simulink model "Table_airbus_v1"  (R2021b)
settings: Solver=VariableStepAuto  StartTime=0.0  StopTime=20  MaxStep=0.01  RelTol=0.01
undefined symbols (not defined in the file): X, Y, Z
libraries: sm_lib x907, fl_lib x69, nesl_utility x53, sdl_lib x10, ee_lib x7, slpidlib x6, simulink x5, simulink_extras x4
(part 17 of 18)

== system Table_airbus_v1/Modèle mécanique/Table/table_1_RIGID/x15060_M_01002_Ens_cadre_Default_1_RIGID/x15060_M_01004_Ens_barre_de_cadre_1_Default_2_RIGID/x15060_M_01042_Barre_transversale_AA_DEFAULT_1_RIGID ==
  ReferenceFrame : sm_lib/Frames and Transforms/Reference Frame
  Solid : sm_lib/Body Elements/File Solid  ExtGeomFileName=15060-M-01042-Barre transversale_AA - DEFAULT_Défaut_sldprt.STL  UnitType=Custom  ExtGeomFileUnits=mm  StepReaderType=HEX  ExportConvexHullGeometry=off  InertiaType=Custom  Mass=0.60250400000000004  MassUnits=kg  CenterOfMass=[0 0 -1.04198e-12]  CenterOfMassUnits=mm  MomentsOfInertia=[20808.599999999999 20753.200000000001 65.337600000000009]  MomentsOfInertiaUnits=kg*mm^2  ProductsOfInertia=[0 0 0]  ProductsOfInertiaUnits=kg*mm^2  BasedOnType=Density  Density=1000  DensityUnits=kg/(m^3)  DoExposeReferenceFrame=on  SerializedFrames=<Frames/>  GraphicType=FromGeometry  MarkerShape=Sphere  MarkerSize=10  MarkerSizeUnits=m  GraphicVisPropType=SimpleVisualProperties  GraphicDiffuseColor=[0.898039 0.917647 0.929412]  GraphicSpecularColor=[0.5 0.5 0.5 1.0]  GraphicAmbientColor=[0.15 0.15 0.15 1.0]  GraphicEmissiveColor=[0.0 0.0 0.0 1.0]  GraphicShininess=75  GraphicOpacity=1
  F : PMIOPort  Side=Left
  connections:
  F/RConn1 -- ReferenceFrame/RConn1 -- Solid/RConn1

== system Table_airbus_v1/Modèle mécanique/Table/table_1_RIGID/x15060_M_01002_Ens_cadre_Default_1_RIGID/x15060_M_01004_Ens_barre_de_cadre_1_Default_2_RIGID/x15060_M_01043_Bride_de_barre_AA_DEFAULT_1_RIGID ==
  ReferenceFrame : sm_lib/Frames and Transforms/Reference Frame
  Solid : sm_lib/Body Elements/File Solid  ExtGeomFileName=15060-M-01043-Bride de barre_AA - DEFAULT_Défaut_sldprt.STL  UnitType=Custom  ExtGeomFileUnits=mm  StepReaderType=HEX  ExportConvexHullGeometry=off  InertiaType=Custom  Mass=0.0646534  MassUnits=kg  CenterOfMass=[0 -0.40050599999999997 5.0587200000000001]  CenterOfMassUnits=mm  MomentsOfInertia=[5.7510300000000001 34.636699999999998 39.315600000000003]  MomentsOfInertiaUnits=kg*mm^2  ProductsOfInertia=[0.038467100000000004 0 0]  ProductsOfInertiaUnits=kg*mm^2  BasedOnType=Density  Density=1000  DensityUnits=kg/(m^3)  DoExposeReferenceFrame=on  SerializedFrames=<Frames/>  GraphicType=FromGeometry  MarkerShape=Sphere  MarkerSize=10  MarkerSizeUnits=m  GraphicVisPropType=SimpleVisualProperties  GraphicDiffuseColor=[0.898039 0.917647 0.929412]  GraphicSpecularColor=[0.5 0.5 0.5 1.0]  GraphicAmbientColor=[0.15 0.15 0.15 1.0]  GraphicEmissiveColor=[0.0 0.0 0.0 1.0]  GraphicShininess=75  GraphicOpacity=1
  F : PMIOPort  Side=Left
  connections:
  F/RConn1 -- ReferenceFrame/RConn1 -- Solid/RConn1

== system Table_airbus_v1/Modèle mécanique/Table/table_1_RIGID/x15060_M_01002_Ens_cadre_Default_1_RIGID/x15060_M_01004_Ens_barre_de_cadre_1_Default_2_RIGID/x15060_M_01043_Bride_de_barre_AA_DEFAULT_2_RIGID ==
  ReferenceFrame : sm_lib/Frames and Transforms/Reference Frame
  Solid : sm_lib/Body Elements/File Solid  ExtGeomFileName=15060-M-01043-Bride de barre_AA - DEFAULT_Défaut_sldprt.STL  UnitType=Custom  ExtGeomFileUnits=mm  StepReaderType=HEX  ExportConvexHullGeometry=off  InertiaType=Custom  Mass=0.0646534  MassUnits=kg  CenterOfMass=[0 -0.40050599999999997 5.0587200000000001]  CenterOfMassUnits=mm  MomentsOfInertia=[5.7510300000000001 34.636699999999998 39.315600000000003]  MomentsOfInertiaUnits=kg*mm^2  ProductsOfInertia=[0.038467100000000004 0 0]  ProductsOfInertiaUnits=kg*mm^2  BasedOnType=Density  Density=1000  DensityUnits=kg/(m^3)  DoExposeReferenceFrame=on  SerializedFrames=<Frames/>  GraphicType=FromGeometry  MarkerShape=Sphere  MarkerSize=10  MarkerSizeUnits=m  GraphicVisPropType=SimpleVisualProperties  GraphicDiffuseColor=[0.898039 0.917647 0.929412]  GraphicSpecularColor=[0.5 0.5 0.5 1.0]  GraphicAmbientColor=[0.15 0.15 0.15 1.0]  GraphicEmissiveColor=[0.0 0.0 0.0 1.0]  GraphicShininess=75  GraphicOpacity=1
  F : PMIOPort  Side=Left
  connections:
  F/RConn1 -- ReferenceFrame/RConn1 -- Solid/RConn1

== system Table_airbus_v1/Modèle mécanique/Table/table_1_RIGID/x15060_M_01002_Ens_cadre_Default_1_RIGID/x15060_M_01004_Ens_barre_de_cadre_1_Default_2_RIGID/x15060_M_01051_Plaquette_sur_glissiere_SYM_AA_DEFAULT_1_RIGID ==
  ReferenceFrame : sm_lib/Frames and Transforms/Reference Frame
  Solid : sm_lib/Body Elements/File Solid  ExtGeomFileName=15060-M-01051-Plaquette sur glissiere - SYM_AA - DEFAULT_Défaut_sldprt.STL  UnitType=Custom  ExtGeomFileUnits=mm  StepReaderType=HEX  ExportConvexHullGeometry=off  InertiaType=Custom  Mass=0.066997100000000004  MassUnits=kg  CenterOfMass=[-1.5299699999999998 -0.085981099999999991 -4.9779900000000001]  CenterOfMassUnits=mm  MomentsOfInertia=[7.6590799999999994 34.768699999999995 41.326299999999996]  MomentsOfInertiaUnits=kg*mm^2  ProductsOfInertia=[0.0011704100000000002 0.039114500000000003 -0.014373]  ProductsOfInertiaUnits=kg*mm^2  BasedOnType=Density  Density=1000  DensityUnits=kg/(m^3)  DoExposeReferenceFrame=on  SerializedFrames=<Frames/>  GraphicType=FromGeometry  MarkerShape=Sphere  MarkerSize=10  MarkerSizeUnits=m  GraphicVisPropType=SimpleVisualProperties  GraphicDiffuseColor=[0.898039 0.917647 0.929412]  GraphicSpecularColor=[0.5 0.5 0.5 1.0]  GraphicAmbientColor=[0.15 0.15 0.15 1.0]  GraphicEmissiveColor=[0.0 0.0 0.0 1.0]  GraphicShininess=75  GraphicOpacity=1
  F : PMIOPort  Side=Left
  connections:
  F/RConn1 -- ReferenceFrame/RConn1 -- Solid/RConn1

== system Table_airbus_v1/Modèle mécanique/Table/table_1_RIGID/x15060_M_01002_Ens_cadre_Default_1_RIGID/x15060_M_01004_Ens_barre_de_cadre_1_Default_2_RIGID/x15060_NLM_Goupille_cyl_3_Lgr_16_03320_03x16_AA_DEFAULT_1_RIGID ==
  ReferenceFrame : sm_lib/Frames and Transforms/Reference Frame
  Solid : sm_lib/Body Elements/File Solid  ExtGeomFileName=15060-NLM-Goupille cyl I3 Lgr 16 - 03320-03x16_AA - DEFAULT_Défaut_sldprt.STL  UnitType=Custom  ExtGeomFileUnits=mm  StepReaderType=HEX  ExportConvexHullGeometry=off  InertiaType=Custom  Mass=0.000113097  MassUnits=kg  CenterOfMass=[8 0 0]  CenterOfMassUnits=mm  MomentsOfInertia=[0.00012723500000000001 0.0024763599999999999 0.0024763599999999999]  MomentsOfInertiaUnits=kg*mm^2  ProductsOfInertia=[0 0 0]  ProductsOfInertiaUnits=kg*mm^2  BasedOnType=Density  Density=1000  DensityUnits=kg/(m^3)  DoExposeReferenceFrame=on  SerializedFrames=<Frames/>  GraphicType=FromGeometry  MarkerShape=Sphere  MarkerSize=10  MarkerSizeUnits=m  GraphicVisPropType=SimpleVisualProperties  GraphicDiffuseColor=[0.792157 0.819608 0.933333]  GraphicSpecularColor=[0.5 0.5 0.5 1.0]  GraphicAmbientColor=[0.15 0.15 0.15 1.0]  GraphicEmissiveColor=[0.0 0.0 0.0 1.0]  GraphicShininess=75  GraphicOpacity=1
  F : PMIOPort  Side=Left
  connections:
  F/RConn1 -- Solid/RConn1 -- ReferenceFrame/RConn1

== system Table_airbus_v1/Modèle mécanique/Table/table_1_RIGID/x15060_M_01002_Ens_cadre_Default_1_RIGID/x15060_M_01004_Ens_barre_de_cadre_1_Default_2_RIGID/x15060_NLM_Goupille_cyl_3_Lgr_16_03320_03x16_AA_DEFAULT_2_RIGID ==
  ReferenceFrame : sm_lib/Frames and Transforms/Reference Frame
  Solid : sm_lib/Body Elements/File Solid  ExtGeomFileName=15060-NLM-Goupille cyl I3 Lgr 16 - 03320-03x16_AA - DEFAULT_Défaut_sldprt.STL  UnitType=Custom  ExtGeomFileUnits=mm  StepReaderType=HEX  ExportConvexHullGeometry=off  InertiaType=Custom  Mass=0.000113097  MassUnits=kg  CenterOfMass=[8 0 0]  CenterOfMassUnits=mm  MomentsOfInertia=[0.00012723500000000001 0.0024763599999999999 0.0024763599999999999]  MomentsOfInertiaUnits=kg*mm^2  ProductsOfInertia=[0 0 0]  ProductsOfInertiaUnits=kg*mm^2  BasedOnType=Density  Density=1000  DensityUnits=kg/(m^3)  DoExposeReferenceFrame=on  SerializedFrames=<Frames/>  GraphicType=FromGeometry  MarkerShape=Sphere  MarkerSize=10  MarkerSizeUnits=m  GraphicVisPropType=SimpleVisualProperties  GraphicDiffuseColor=[0.792157 0.819608 0.933333]  GraphicSpecularColor=[0.5 0.5 0.5 1.0]  GraphicAmbientColor=[0.15 0.15 0.15 1.0]  GraphicEmissiveColor=[0.0 0.0 0.0 1.0]  GraphicShininess=75  GraphicOpacity=1
  F : PMIOPort  Side=Left
  connections:
  F/RConn1 -- Solid/RConn1 -- ReferenceFrame/RConn1

== system Table_airbus_v1/Modèle mécanique/Table/table_1_RIGID/x15060_M_01002_Ens_cadre_Default_1_RIGID/x15060_M_01004_Ens_barre_de_cadre_1_Default_2_RIGID/x15060_NLM_Poign_e_Miniwing_M6_06652_006_X_15_1_RIGID ==
  ReferenceFrame : sm_lib/Frames and Transforms/Reference Frame
  Solid : sm_lib/Body Elements/File Solid  ExtGeomFileName=15060-NLM-Poignee Miniwing M6 - 06652-006 X 15_Défaut_sldprt.STL  UnitType=Custom  ExtGeomFileUnits=mm  StepReaderType=HEX  ExportConvexHullGeometry=off  InertiaType=Custom  Mass=0.0031415499999999999  MassUnits=kg  CenterOfMass=[0 5.4933500000000004 0]  CenterOfMassUnits=mm  MomentsOfInertia=[0.151592 0.116684 0.22078500000000001]  MomentsOfInertiaUnits=kg*mm^2  ProductsOfInertia=[0 0.0064548499999999998 0]  ProductsOfInertiaUnits=kg*mm^2  BasedOnType=Density  Density=1000  DensityUnits=kg/(m^3)  DoExposeReferenceFrame=on  SerializedFrames=<Frames/>  GraphicType=FromGeometry  MarkerShape=Sphere  MarkerSize=10  MarkerSizeUnits=m  GraphicVisPropType=SimpleVisualProperties  GraphicDiffuseColor=[0.792157 0.819608 0.933333]  GraphicSpecularColor=[0.5 0.5 0.5 1.0]  GraphicAmbientColor=[0.15 0.15 0.15 1.0]  GraphicEmissiveColor=[0.0 0.0 0.0 1.0]  GraphicShininess=75  GraphicOpacity=1
  F : PMIOPort  Side=Left
  connections:
  F/RConn1 -- Solid/RConn1 -- ReferenceFrame/RConn1

== system Table_airbus_v1/Modèle mécanique/Table/table_1_RIGID/x15060_M_01002_Ens_cadre_Default_1_RIGID/x15060_M_01004_Ens_barre_de_cadre_1_Default_2_RIGID/x15060_NLM_Poign_e_Miniwing_M6_06652_006_X_15_2_RIGID ==
  ReferenceFrame : sm_lib/Frames and Transforms/Reference Frame
  Solid : sm_lib/Body Elements/File Solid  ExtGeomFileName=15060-NLM-Poignee Miniwing M6 - 06652-006 X 15_Défaut_sldprt.STL  UnitType=Custom  ExtGeomFileUnits=mm  StepReaderType=HEX  ExportConvexHullGeometry=off  InertiaType=Custom  Mass=0.0031415499999999999  MassUnits=kg  CenterOfMass=[0 5.4933500000000004 0]  CenterOfMassUnits=mm  MomentsOfInertia=[0.151592 0.116684 0.22078500000000001]  MomentsOfInertiaUnits=kg*mm^2  ProductsOfInertia=[0 0.0064548499999999998 0]  ProductsOfInertiaUnits=kg*mm^2  BasedOnType=Density  Density=1000  DensityUnits=kg/(m^3)  DoExposeReferenceFrame=on  SerializedFrames=<Frames/>  GraphicType=FromGeometry  MarkerShape=Sphere  MarkerSize=10  MarkerSizeUnits=m  GraphicVisPropType=SimpleVisualProperties  GraphicDiffuseColor=[0.792157 0.819608 0.933333]  GraphicSpecularColor=[0.5 0.5 0.5 1.0]  GraphicAmbientColor=[0.15 0.15 0.15 1.0]  GraphicEmissiveColor=[0.0 0.0 0.0 1.0]  GraphicShininess=75  GraphicOpacity=1
  F : PMIOPort  Side=Left
  connections:
  F/RConn1 -- Solid/RConn1 -- ReferenceFrame/RConn1

== system Table_airbus_v1/Modèle mécanique/Table/table_1_RIGID/x15060_M_01002_Ens_cadre_Default_1_RIGID/x15060_M_01004_Ens_barre_de_cadre_1_Default_2_RIGID/x15060_Rondelle_Rondelle_Etroite_Z_4_1_RIGID ==
  ReferenceFrame : sm_lib/Frames and Transforms/Reference Frame
  Solid : sm_lib/Body Elements/File Solid  ExtGeomFileName=15060-Rondelle-_Rondelle Etroite Z 4_Défaut_sldprt.STL  UnitType=Custom  ExtGeomFileUnits=mm  StepReaderType=HEX  ExportConvexHullGeometry=off  InertiaType=Custom  Mass=3.9276200000000002e-05  MassUnits=kg  CenterOfMass=[0 0.40000000000000002 0]  CenterOfMassUnits=mm  MomentsOfInertia=[0.000246319 0.00048844899999999996 0.000246319]  MomentsOfInertiaUnits=kg*mm^2  ProductsOfInertia=[0 0 0]  ProductsOfInertiaUnits=kg*mm^2  BasedOnType=Density  Density=1000  DensityUnits=kg/(m^3)  DoExposeReferenceFrame=on  SerializedFrames=<Frames/>  GraphicType=FromGeometry  MarkerShape=Sphere  MarkerSize=10  MarkerSizeUnits=m  GraphicVisPropType=SimpleVisualProperties  GraphicDiffuseColor=[0.792157 0.819608 0.933333]  GraphicSpecularColor=[0.5 0.5 0.5 1.0]  GraphicAmbientColor=[0.15 0.15 0.15 1.0]  GraphicEmissiveColor=[0.0 0.0 0.0 1.0]  GraphicShininess=75  GraphicOpacity=1
  F : PMIOPort  Side=Left
  connections:
  F/RConn1 -- ReferenceFrame/RConn1 -- Solid/RConn1

== system Table_airbus_v1/Modèle mécanique/Table/table_1_RIGID/x15060_M_01002_Ens_cadre_Default_1_RIGID/x15060_M_01004_Ens_barre_de_cadre_1_Default_2_RIGID/x15060_Rondelle_Rondelle_Etroite_Z_4_2_RIGID ==
  ReferenceFrame : sm_lib/Frames and Transforms/Reference Frame
  Solid : sm_lib/Body Elements/File Solid  ExtGeomFileName=15060-Rondelle-_Rondelle Etroite Z 4_Défaut_sldprt.STL  UnitType=Custom  ExtGeomFileUnits=mm  StepReaderType=HEX  ExportConvexHullGeometry=off  InertiaType=Custom  Mass=3.9276200000000002e-05  MassUnits=kg  CenterOfMass=[0 0.40000000000000002 0]  CenterOfMassUnits=mm  MomentsOfInertia=[0.000246319 0.00048844899999999996 0.000246319]  MomentsOfInertiaUnits=kg*mm^2  ProductsOfInertia=[0 0 0]  ProductsOfInertiaUnits=kg*mm^2  BasedOnType=Density  Density=1000  DensityUnits=kg/(m^3)  DoExposeReferenceFrame=on  SerializedFrames=<Frames/>  GraphicType=FromGeometry  MarkerShape=Sphere  MarkerSize=10  MarkerSizeUnits=m  GraphicVisPropType=SimpleVisualProperties  GraphicDiffuseColor=[0.792157 0.819608 0.933333]  GraphicSpecularColor=[0.5 0.5 0.5 1.0]  GraphicAmbientColor=[0.15 0.15 0.15 1.0]  GraphicEmissiveColor=[0.0 0.0 0.0 1.0]  GraphicShininess=75  GraphicOpacity=1
  F : PMIOPort  Side=Left
  connections:
  F/RConn1 -- ReferenceFrame/RConn1 -- Solid/RConn1

== system Table_airbus_v1/Modèle mécanique/Table/table_1_RIGID/x15060_M_01002_Ens_cadre_Default_1_RIGID/x15060_M_01004_Ens_barre_de_cadre_1_Default_2_RIGID/x15060_Rondelle_Rondelle_Etroite_Z_4_3_RIGID ==
  ReferenceFrame : sm_lib/Frames and Transforms/Reference Frame
  Solid : sm_lib/Body Elements/File Solid  ExtGeomFileName=15060-Rondelle-_Rondelle Etroite Z 4_Défaut_sldprt.STL  UnitType=Custom  ExtGeomFileUnits=mm  StepReaderType=HEX  ExportConvexHullGeometry=off  InertiaType=Custom  Mass=3.9276200000000002e-05  MassUnits=kg  CenterOfMass=[0 0.40000000000000002 0]  CenterOfMassUnits=mm  MomentsOfInertia=[0.000246319 0.00048844899999999996 0.000246319]  MomentsOfInertiaUnits=kg*mm^2  ProductsOfInertia=[0 0 0]  ProductsOfInertiaUnits=kg*mm^2  BasedOnType=Density  Density=1000  DensityUnits=kg/(m^3)  DoExposeReferenceFrame=on  SerializedFrames=<Frames/>  GraphicType=FromGeometry  MarkerShape=Sphere  MarkerSize=10  MarkerSizeUnits=m  GraphicVisPropType=SimpleVisualProperties  GraphicDiffuseColor=[0.792157 0.819608 0.933333]  GraphicSpecularColor=[0.5 0.5 0.5 1.0]  GraphicAmbientColor=[0.15 0.15 0.15 1.0]  GraphicEmissiveColor=[0.0 0.0 0.0 1.0]  GraphicShininess=75  GraphicOpacity=1
  F : PMIOPort  Side=Left
  connections:
  F/RConn1 -- ReferenceFrame/RConn1 -- Solid/RConn1

== system Table_airbus_v1/Modèle mécanique/Table/table_1_RIGID/x15060_M_01002_Ens_cadre_Default_1_RIGID/x15060_M_01004_Ens_barre_de_cadre_1_Default_2_RIGID/x15060_Vis_CHc_vis_CHc_M_4_X_12_1_RIGID ==
  ReferenceFrame : sm_lib/Frames and Transforms/Reference Frame
  Solid : sm_lib/Body Elements/File Solid  ExtGeomFileName="15060-Vis CHc-_vis CHc M 4 X  12_Défaut_sldprt.STL"  UnitType=Custom  ExtGeomFileUnits=mm  StepReaderType=HEX  ExportConvexHullGeometry=off  InertiaType=Custom  Mass=0.00028164600000000003  MassUnits=kg  CenterOfMass=[0 1.2813e-08 6.3179499999999997]  CenterOfMassUnits=mm  MomentsOfInertia=[0.0068365400000000003 0.0068372900000000002 0.00118534]  MomentsOfInertiaUnits=kg*mm^2  ProductsOfInertia=[0 0 -4.9500699999999998e-08]  ProductsOfInertiaUnits=kg*mm^2  BasedOnType=Density  Density=1000  DensityUnits=kg/(m^3)  DoExposeReferenceFrame=on  SerializedFrames=<Frames/>  GraphicType=FromGeometry  MarkerShape=Sphere  MarkerSize=10  MarkerSizeUnits=m  GraphicVisPropType=SimpleVisualProperties  GraphicDiffuseColor=[0.792157 0.819608 0.933333]  GraphicSpecularColor=[0.5 0.5 0.5 1.0]  GraphicAmbientColor=[0.15 0.15 0.15 1.0]  GraphicEmissiveColor=[0.0 0.0 0.0 1.0]  GraphicShininess=75  GraphicOpacity=1
  F : PMIOPort  Side=Left
  connections:
  F/RConn1 -- ReferenceFrame/RConn1 -- Solid/RConn1

== system Table_airbus_v1/Modèle mécanique/Table/table_1_RIGID/x15060_M_01002_Ens_cadre_Default_1_RIGID/x15060_M_01004_Ens_barre_de_cadre_1_Default_2_RIGID/x15060_Vis_CHc_vis_CHc_M_4_X_16_1_RIGID ==
  ReferenceFrame : sm_lib/Frames and Transforms/Reference Frame
  Solid : sm_lib/Body Elements/File Solid  ExtGeomFileName="15060-Vis CHc-_vis CHc M 4 X  16_Défaut_sldprt.STL"  UnitType=Custom  ExtGeomFileUnits=mm  StepReaderType=HEX  ExportConvexHullGeometry=off  InertiaType=Custom  Mass=0.00033190900000000002  MassUnits=kg  CenterOfMass=[0 1.06986e-08 8.0784000000000002]  CenterOfMassUnits=mm  MomentsOfInertia=[0.0127177 0.0127186 0.00128578]  MomentsOfInertiaUnits=kg*mm^2  ProductsOfInertia=[0 0 -6.1878200000000004e-08]  ProductsOfInertiaUnits=kg*mm^2  BasedOnType=Density  Density=1000  DensityUnits=kg/(m^3)  DoExposeReferenceFrame=on  SerializedFrames=<Frames/>  GraphicType=FromGeometry  MarkerShape=Sphere  MarkerSize=10  MarkerSizeUnits=m  GraphicVisPropType=SimpleVisualProperties  GraphicDiffuseColor=[0.792157 0.819608 0.933333]  GraphicSpecularColor=[0.5 0.5 0.5 1.0]  GraphicAmbientColor=[0.15 0.15 0.15 1.0]  GraphicEmissiveColor=[0.0 0.0 0.0 1.0]  GraphicShininess=75  GraphicOpacity=1
  F : PMIOPort  Side=Left
  connections:
  F/RConn1 -- ReferenceFrame/RConn1 -- Solid/RConn1

== system Table_airbus_v1/Modèle mécanique/Table/table_1_RIGID/x15060_M_01002_Ens_cadre_Default_1_RIGID/x15060_M_01005_Ens_barre_de_cadre_2_Default_1_RIGID/x15060_M_01029_Plaquette_haute_sur_glissiere_AA_DEFAULT_1_RIGID ==
  ReferenceFrame : sm_lib/Frames and Transforms/Reference Frame
  Solid : sm_lib/Body Elements/File Solid  ExtGeomFileName=15060-M-01029-Plaquette haute sur glissiere_AA - DEFAULT_Défaut_sldprt.STL  UnitType=Custom  ExtGeomFileUnits=mm  StepReaderType=HEX  ExportConvexHullGeometry=off  InertiaType=Custom  Mass=0.16431999999999999  MassUnits=kg  CenterOfMass=[-0.63256999999999997 23.438800000000001 4.9895300000000002]  CenterOfMassUnits=mm  MomentsOfInertia=[87.900999999999996 87.570599999999999 172.749]  MomentsOfInertiaUnits=kg*mm^2  ProductsOfInertia=[0.0346898 -0.044105600000000002 2.4036900000000001]  ProductsOfInertiaUnits=kg*mm^2  BasedOnType=Density  Density=1000  DensityUnits=kg/(m^3)  DoExposeReferenceFrame=on  SerializedFrames=<Frames/>  GraphicType=FromGeometry  MarkerShape=Sphere  MarkerSize=10  MarkerSizeUnits=m  GraphicVisPropType=SimpleVisualProperties  GraphicDiffuseColor=[0.898039 0.917647 0.929412]  GraphicSpecularColor=[0.5 0.5 0.5 1.0]  GraphicAmbientColor=[0.15 0.15 0.15 1.0]  GraphicEmissiveColor=[0.0 0.0 0.0 1.0]  GraphicShininess=75  GraphicOpacity=1
  F : PMIOPort  Side=Left
  connections:
  F/RConn1 -- ReferenceFrame/RConn1 -- Solid/RConn1

== system Table_airbus_v1/Modèle mécanique/Table/table_1_RIGID/x15060_M_01002_Ens_cadre_Default_1_RIGID/x15060_M_01005_Ens_barre_de_cadre_2_Default_1_RIGID/x15060_M_01042_Barre_transversale_AA_DEFAULT_1_RIGID ==
  ReferenceFrame : sm_lib/Frames and Transforms/Reference Frame
  Solid : sm_lib/Body Elements/File Solid  ExtGeomFileName=15060-M-01042-Barre transversale_AA - DEFAULT_Défaut_sldprt.STL  UnitType=Custom  ExtGeomFileUnits=mm  StepReaderType=HEX  ExportConvexHullGeometry=off  InertiaType=Custom  Mass=0.60250400000000004  MassUnits=kg  CenterOfMass=[0 0 -1.04198e-12]  CenterOfMassUnits=mm  MomentsOfInertia=[20808.599999999999 20753.200000000001 65.337600000000009]  MomentsOfInertiaUnits=kg*mm^2  ProductsOfInertia=[0 0 0]  ProductsOfInertiaUnits=kg*mm^2  BasedOnType=Density  Density=1000  DensityUnits=kg/(m^3)  DoExposeReferenceFrame=on  SerializedFrames=<Frames/>  GraphicType=FromGeometry  MarkerShape=Sphere  MarkerSize=10  MarkerSizeUnits=m  GraphicVisPropType=SimpleVisualProperties  GraphicDiffuseColor=[0.898039 0.917647 0.929412]  GraphicSpecularColor=[0.5 0.5 0.5 1.0]  GraphicAmbientColor=[0.15 0.15 0.15 1.0]  GraphicEmissiveColor=[0.0 0.0 0.0 1.0]  GraphicShininess=75  GraphicOpacity=1
  F : PMIOPort  Side=Left
  connections:
  F/RConn1 -- ReferenceFrame/RConn1 -- Solid/RConn1

== system Table_airbus_v1/Modèle mécanique/Table/table_1_RIGID/x15060_M_01002_Ens_cadre_Default_1_RIGID/x15060_M_01005_Ens_barre_de_cadre_2_Default_1_RIGID/x15060_M_01043_Bride_de_barre_AA_DEFAULT_1_RIGID ==
  ReferenceFrame : sm_lib/Frames and Transforms/Reference Frame
  Solid : sm_lib/Body Elements/File Solid  ExtGeomFileName=15060-M-01043-Bride de barre_AA - DEFAULT_Défaut_sldprt.STL  UnitType=Custom  ExtGeomFileUnits=mm  StepReaderType=HEX  ExportConvexHullGeometry=off  InertiaType=Custom  Mass=0.0646534  MassUnits=kg  CenterOfMass=[0 -0.40050599999999997 5.0587200000000001]  CenterOfMassUnits=mm  MomentsOfInertia=[5.7510300000000001 34.636699999999998 39.315600000000003]  MomentsOfInertiaUnits=kg*mm^2  ProductsOfInertia=[0.038467100000000004 0 0]  ProductsOfInertiaUnits=kg*mm^2  BasedOnType=Density  Density=1000  DensityUnits=kg/(m^3)  DoExposeReferenceFrame=on  SerializedFrames=<Frames/>  GraphicType=FromGeometry  MarkerShape=Sphere  MarkerSize=10  MarkerSizeUnits=m  GraphicVisPropType=SimpleVisualProperties  GraphicDiffuseColor=[0.898039 0.917647 0.929412]  GraphicSpecularColor=[0.5 0.5 0.5 1.0]  GraphicAmbientColor=[0.15 0.15 0.15 1.0]  GraphicEmissiveColor=[0.0 0.0 0.0 1.0]  GraphicShininess=75  GraphicOpacity=1
  F : PMIOPort  Side=Left
  connections:
  F/RConn1 -- ReferenceFrame/RConn1 -- Solid/RConn1

== system Table_airbus_v1/Modèle mécanique/Table/table_1_RIGID/x15060_M_01002_Ens_cadre_Default_1_RIGID/x15060_M_01005_Ens_barre_de_cadre_2_Default_1_RIGID/x15060_M_01043_Bride_de_barre_AA_DEFAULT_2_RIGID ==
  ReferenceFrame : sm_lib/Frames and Transforms/Reference Frame
  Solid : sm_lib/Body Elements/File Solid  ExtGeomFileName=15060-M-01043-Bride de barre_AA - DEFAULT_Défaut_sldprt.STL  UnitType=Custom  ExtGeomFileUnits=mm  StepReaderType=HEX  ExportConvexHullGeometry=off  InertiaType=Custom  Mass=0.0646534  MassUnits=kg  CenterOfMass=[0 -0.40050599999999997 5.0587200000000001]  CenterOfMassUnits=mm  MomentsOfInertia=[5.7510300000000001 34.636699999999998 39.315600000000003]  MomentsOfInertiaUnits=kg*mm^2  ProductsOfInertia=[0.038467100000000004 0 0]  ProductsOfInertiaUnits=kg*mm^2  BasedOnType=Density  Density=1000  DensityUnits=kg/(m^3)  DoExposeReferenceFrame=on  SerializedFrames=<Frames/>  GraphicType=FromGeometry  MarkerShape=Sphere  MarkerSize=10  MarkerSizeUnits=m  GraphicVisPropType=SimpleVisualProperties  GraphicDiffuseColor=[0.898039 0.917647 0.929412]  GraphicSpecularColor=[0.5 0.5 0.5 1.0]  GraphicAmbientColor=[0.15 0.15 0.15 1.0]  GraphicEmissiveColor=[0.0 0.0 0.0 1.0]  GraphicShininess=75  GraphicOpacity=1
  F : PMIOPort  Side=Left
  connections:
  F/RConn1 -- ReferenceFrame/RConn1 -- Solid/RConn1

== system Table_airbus_v1/Modèle mécanique/Table/table_1_RIGID/x15060_M_01002_Ens_cadre_Default_1_RIGID/x15060_M_01005_Ens_barre_de_cadre_2_Default_1_RIGID/x15060_M_01053_Plaquette_haute_sur_glissiere_SYM_AA_DEFAULT_1_R ==
  ReferenceFrame : sm_lib/Frames and Transforms/Reference Frame
  Solid : sm_lib/Body Elements/File Solid  ExtGeomFileName=15060-M-01053-Plaquette haute sur glissiere - SYM_AA - DEFAULT_Défaut_sldprt.STL  UnitType=Custom  ExtGeomFileUnits=mm  StepReaderType=HEX  ExportConvexHullGeometry=off  InertiaType=Custom  Mass=0.16431999999999999  MassUnits=kg  CenterOfMass=[-0.632606 23.438800000000001 -4.9895300000000002]  CenterOfMassUnits=mm  MomentsOfInertia=[87.900800000000004 87.570599999999999 172.749]  MomentsOfInertiaUnits=kg*mm^2  ProductsOfInertia=[-0.0346886 0.044093199999999999 2.4038600000000003]  ProductsOfInertiaUnits=kg*mm^2  BasedOnType=Density  Density=1000  DensityUnits=kg/(m^3)  DoExposeReferenceFrame=on  SerializedFrames=<Frames/>  GraphicType=FromGeometry  MarkerShape=Sphere  MarkerSize=10  MarkerSizeUnits=m  GraphicVisPropType=SimpleVisualProperties  GraphicDiffuseColor=[0.898039 0.917647 0.929412]  GraphicSpecularColor=[0.5 0.5 0.5 1.0]  GraphicAmbientColor=[0.15 0.15 0.15 1.0]  GraphicEmissiveColor=[0.0 0.0 0.0 1.0]  GraphicShininess=75  GraphicOpacity=1
  F : PMIOPort  Side=Left
  connections:
  F/RConn1 -- ReferenceFrame/RConn1 -- Solid/RConn1

== system Table_airbus_v1/Modèle mécanique/Table/table_1_RIGID/x15060_M_01002_Ens_cadre_Default_1_RIGID/x15060_M_01005_Ens_barre_de_cadre_2_Default_1_RIGID/x15060_NLM_Goupille_cyl_3_Lgr_16_03320_03x16_AA_DEFAULT_1_RIGID ==
  ReferenceFrame : sm_lib/Frames and Transforms/Reference Frame
  Solid : sm_lib/Body Elements/File Solid  ExtGeomFileName=15060-NLM-Goupille cyl I3 Lgr 16 - 03320-03x16_AA - DEFAULT_Défaut_sldprt.STL  UnitType=Custom  ExtGeomFileUnits=mm  StepReaderType=HEX  ExportConvexHullGeometry=off  InertiaType=Custom  Mass=0.000113097  MassUnits=kg  CenterOfMass=[8 0 0]  CenterOfMassUnits=mm  MomentsOfInertia=[0.00012723500000000001 0.0024763599999999999 0.0024763599999999999]  MomentsOfInertiaUnits=kg*mm^2  ProductsOfInertia=[0 0 0]  ProductsOfInertiaUnits=kg*mm^2  BasedOnType=Density  Density=1000  DensityUnits=kg/(m^3)  DoExposeReferenceFrame=on  SerializedFrames=<Frames/>  GraphicType=FromGeometry  MarkerShape=Sphere  MarkerSize=10  MarkerSizeUnits=m  GraphicVisPropType=SimpleVisualProperties  GraphicDiffuseColor=[0.792157 0.819608 0.933333]  GraphicSpecularColor=[0.5 0.5 0.5 1.0]  GraphicAmbientColor=[0.15 0.15 0.15 1.0]  GraphicEmissiveColor=[0.0 0.0 0.0 1.0]  GraphicShininess=75  GraphicOpacity=1
  F : PMIOPort  Side=Left
  connections:
  F/RConn1 -- Solid/RConn1 -- ReferenceFrame/RConn1

== system Table_airbus_v1/Modèle mécanique/Table/table_1_RIGID/x15060_M_01002_Ens_cadre_Default_1_RIGID/x15060_M_01005_Ens_barre_de_cadre_2_Default_1_RIGID/x15060_NLM_Goupille_cyl_3_Lgr_16_03320_03x16_AA_DEFAULT_2_RIGID ==
  ReferenceFrame : sm_lib/Frames and Transforms/Reference Frame
  Solid : sm_lib/Body Elements/File Solid  ExtGeomFileName=15060-NLM-Goupille cyl I3 Lgr 16 - 03320-03x16_AA - DEFAULT_Défaut_sldprt.STL  UnitType=Custom  ExtGeomFileUnits=mm  StepReaderType=HEX  ExportConvexHullGeometry=off  InertiaType=Custom  Mass=0.000113097  MassUnits=kg  CenterOfMass=[8 0 0]  CenterOfMassUnits=mm  MomentsOfInertia=[0.00012723500000000001 0.0024763599999999999 0.0024763599999999999]  MomentsOfInertiaUnits=kg*mm^2  ProductsOfInertia=[0 0 0]  ProductsOfInertiaUnits=kg*mm^2  BasedOnType=Density  Density=1000  DensityUnits=kg/(m^3)  DoExposeReferenceFrame=on  SerializedFrames=<Frames/>  GraphicType=FromGeometry  MarkerShape=Sphere  MarkerSize=10  MarkerSizeUnits=m  GraphicVisPropType=SimpleVisualProperties  GraphicDiffuseColor=[0.792157 0.819608 0.933333]  GraphicSpecularColor=[0.5 0.5 0.5 1.0]  GraphicAmbientColor=[0.15 0.15 0.15 1.0]  GraphicEmissiveColor=[0.0 0.0 0.0 1.0]  GraphicShininess=75  GraphicOpacity=1
  F : PMIOPort  Side=Left
  connections:
  F/RConn1 -- Solid/RConn1 -- ReferenceFrame/RConn1

== system Table_airbus_v1/Modèle mécanique/Table/table_1_RIGID/x15060_M_01002_Ens_cadre_Default_1_RIGID/x15060_M_01005_Ens_barre_de_cadre_2_Default_1_RIGID/x15060_NLM_Poign_e_Miniwing_M6_06652_006_X_15_1_RIGID ==
  ReferenceFrame : sm_lib/Frames and Transforms/Reference Frame
  Solid : sm_lib/Body Elements/File Solid  ExtGeomFileName=15060-NLM-Poignee Miniwing M6 - 06652-006 X 15_Défaut_sldprt.STL  UnitType=Custom  ExtGeomFileUnits=mm  StepReaderType=HEX  ExportConvexHullGeometry=off  InertiaType=Custom  Mass=0.0031415499999999999  MassUnits=kg  CenterOfMass=[0 5.4933500000000004 0]  CenterOfMassUnits=mm  MomentsOfInertia=[0.151592 0.116684 0.22078500000000001]  MomentsOfInertiaUnits=kg*mm^2  ProductsOfInertia=[0 0.0064548499999999998 0]  ProductsOfInertiaUnits=kg*mm^2  BasedOnType=Density  Density=1000  DensityUnits=kg/(m^3)  DoExposeReferenceFrame=on  SerializedFrames=<Frames/>  GraphicType=FromGeometry  MarkerShape=Sphere  MarkerSize=10  MarkerSizeUnits=m  GraphicVisPropType=SimpleVisualProperties  GraphicDiffuseColor=[0.792157 0.819608 0.933333]  GraphicSpecularColor=[0.5 0.5 0.5 1.0]  GraphicAmbientColor=[0.15 0.15 0.15 1.0]  GraphicEmissiveColor=[0.0 0.0 0.0 1.0]  GraphicShininess=75  GraphicOpacity=1
  F : PMIOPort  Side=Left
  connections:
  F/RConn1 -- Solid/RConn1 -- ReferenceFrame/RConn1

== system Table_airbus_v1/Modèle mécanique/Table/table_1_RIGID/x15060_M_01002_Ens_cadre_Default_1_RIGID/x15060_M_01005_Ens_barre_de_cadre_2_Default_1_RIGID/x15060_NLM_Poign_e_Miniwing_M6_06652_006_X_15_2_RIGID ==
  ReferenceFrame : sm_lib/Frames and Transforms/Reference Frame
  Solid : sm_lib/Body Elements/File Solid  ExtGeomFileName=15060-NLM-Poignee Miniwing M6 - 06652-006 X 15_Défaut_sldprt.STL  UnitType=Custom  ExtGeomFileUnits=mm  StepReaderType=HEX  ExportConvexHullGeometry=off  InertiaType=Custom  Mass=0.0031415499999999999  MassUnits=kg  CenterOfMass=[0 5.4933500000000004 0]  CenterOfMassUnits=mm  MomentsOfInertia=[0.151592 0.116684 0.22078500000000001]  MomentsOfInertiaUnits=kg*mm^2  ProductsOfInertia=[0 0.0064548499999999998 0]  ProductsOfInertiaUnits=kg*mm^2  BasedOnType=Density  Density=1000  DensityUnits=kg/(m^3)  DoExposeReferenceFrame=on  SerializedFrames=<Frames/>  GraphicType=FromGeometry  MarkerShape=Sphere  MarkerSize=10  MarkerSizeUnits=m  GraphicVisPropType=SimpleVisualProperties  GraphicDiffuseColor=[0.792157 0.819608 0.933333]  GraphicSpecularColor=[0.5 0.5 0.5 1.0]  GraphicAmbientColor=[0.15 0.15 0.15 1.0]  GraphicEmissiveColor=[0.0 0.0 0.0 1.0]  GraphicShininess=75  GraphicOpacity=1
  F : PMIOPort  Side=Left
  connections:
  F/RConn1 -- Solid/RConn1 -- ReferenceFrame/RConn1

== system Table_airbus_v1/Modèle mécanique/Table/table_1_RIGID/x15060_M_01002_Ens_cadre_Default_1_RIGID/x15060_M_01005_Ens_barre_de_cadre_2_Default_1_RIGID/x15060_Rondelle_Rondelle_Etroite_Z_4_1_RIGID ==
  ReferenceFrame : sm_lib/Frames and Transforms/Reference Frame
  Solid : sm_lib/Body Elements/File Solid  ExtGeomFileName=15060-Rondelle-_Rondelle Etroite Z 4_Défaut_sldprt.STL  UnitType=Custom  ExtGeomFileUnits=mm  StepReaderType=HEX  ExportConvexHullGeometry=off  InertiaType=Custom  Mass=3.9276200000000002e-05  MassUnits=kg  CenterOfMass=[0 0.40000000000000002 0]  CenterOfMassUnits=mm  MomentsOfInertia=[0.000246319 0.00048844899999999996 0.000246319]  MomentsOfInertiaUnits=kg*mm^2  ProductsOfInertia=[0 0 0]  ProductsOfInertiaUnits=kg*mm^2  BasedOnType=Density  Density=1000  DensityUnits=kg/(m^3)  DoExposeReferenceFrame=on  SerializedFrames=<Frames/>  GraphicType=FromGeometry  MarkerShape=Sphere  MarkerSize=10  MarkerSizeUnits=m  GraphicVisPropType=SimpleVisualProperties  GraphicDiffuseColor=[0.792157 0.819608 0.933333]  GraphicSpecularColor=[0.5 0.5 0.5 1.0]  GraphicAmbientColor=[0.15 0.15 0.15 1.0]  GraphicEmissiveColor=[0.0 0.0 0.0 1.0]  GraphicShininess=75  GraphicOpacity=1
  F : PMIOPort  Side=Left
  connections:
  F/RConn1 -- ReferenceFrame/RConn1 -- Solid/RConn1

== system Table_airbus_v1/Modèle mécanique/Table/table_1_RIGID/x15060_M_01002_Ens_cadre_Default_1_RIGID/x15060_M_01005_Ens_barre_de_cadre_2_Default_1_RIGID/x15060_Rondelle_Rondelle_Etroite_Z_4_2_RIGID ==
  ReferenceFrame : sm_lib/Frames and Transforms/Reference Frame
  Solid : sm_lib/Body Elements/File Solid  ExtGeomFileName=15060-Rondelle-_Rondelle Etroite Z 4_Défaut_sldprt.STL  UnitType=Custom  ExtGeomFileUnits=mm  StepReaderType=HEX  ExportConvexHullGeometry=off  InertiaType=Custom  Mass=3.9276200000000002e-05  MassUnits=kg  CenterOfMass=[0 0.40000000000000002 0]  CenterOfMassUnits=mm  MomentsOfInertia=[0.000246319 0.00048844899999999996 0.000246319]  MomentsOfInertiaUnits=kg*mm^2  ProductsOfInertia=[0 0 0]  ProductsOfInertiaUnits=kg*mm^2  BasedOnType=Density  Density=1000  DensityUnits=kg/(m^3)  DoExposeReferenceFrame=on  SerializedFrames=<Frames/>  GraphicType=FromGeometry  MarkerShape=Sphere  MarkerSize=10  MarkerSizeUnits=m  GraphicVisPropType=SimpleVisualProperties  GraphicDiffuseColor=[0.792157 0.819608 0.933333]  GraphicSpecularColor=[0.5 0.5 0.5 1.0]  GraphicAmbientColor=[0.15 0.15 0.15 1.0]  GraphicEmissiveColor=[0.0 0.0 0.0 1.0]  GraphicShininess=75  GraphicOpacity=1
  F : PMIOPort  Side=Left
  connections:
  F/RConn1 -- ReferenceFrame/RConn1 -- Solid/RConn1

== system Table_airbus_v1/Modèle mécanique/Table/table_1_RIGID/x15060_M_01002_Ens_cadre_Default_1_RIGID/x15060_M_01005_Ens_barre_de_cadre_2_Default_1_RIGID/x15060_Rondelle_Rondelle_Etroite_Z_4_3_RIGID ==
  ReferenceFrame : sm_lib/Frames and Transforms/Reference Frame
  Solid : sm_lib/Body Elements/File Solid  ExtGeomFileName=15060-Rondelle-_Rondelle Etroite Z 4_Défaut_sldprt.STL  UnitType=Custom  ExtGeomFileUnits=mm  StepReaderType=HEX  ExportConvexHullGeometry=off  InertiaType=Custom  Mass=3.9276200000000002e-05  MassUnits=kg  CenterOfMass=[0 0.40000000000000002 0]  CenterOfMassUnits=mm  MomentsOfInertia=[0.000246319 0.00048844899999999996 0.000246319]  MomentsOfInertiaUnits=kg*mm^2  ProductsOfInertia=[0 0 0]  ProductsOfInertiaUnits=kg*mm^2  BasedOnType=Density  Density=1000  DensityUnits=kg/(m^3)  DoExposeReferenceFrame=on  SerializedFrames=<Frames/>  GraphicType=FromGeometry  MarkerShape=Sphere  MarkerSize=10  MarkerSizeUnits=m  GraphicVisPropType=SimpleVisualProperties  GraphicDiffuseColor=[0.792157 0.819608 0.933333]  GraphicSpecularColor=[0.5 0.5 0.5 1.0]  GraphicAmbientColor=[0.15 0.15 0.15 1.0]  GraphicEmissiveColor=[0.0 0.0 0.0 1.0]  GraphicShininess=75  GraphicOpacity=1
  F : PMIOPort  Side=Left
  connections:
  F/RConn1 -- ReferenceFrame/RConn1 -- Solid/RConn1

== system Table_airbus_v1/Modèle mécanique/Table/table_1_RIGID/x15060_M_01002_Ens_cadre_Default_1_RIGID/x15060_M_01005_Ens_barre_de_cadre_2_Default_2_RIGID/x15060_M_01029_Plaquette_haute_sur_glissiere_AA_DEFAULT_1_RIGID ==
  ReferenceFrame : sm_lib/Frames and Transforms/Reference Frame
  Solid : sm_lib/Body Elements/File Solid  ExtGeomFileName=15060-M-01029-Plaquette haute sur glissiere_AA - DEFAULT_Défaut_sldprt.STL  UnitType=Custom  ExtGeomFileUnits=mm  StepReaderType=HEX  ExportConvexHullGeometry=off  InertiaType=Custom  Mass=0.16431999999999999  MassUnits=kg  CenterOfMass=[-0.63256999999999997 23.438800000000001 4.9895300000000002]  CenterOfMassUnits=mm  MomentsOfInertia=[87.900999999999996 87.570599999999999 172.749]  MomentsOfInertiaUnits=kg*mm^2  ProductsOfInertia=[0.0346898 -0.044105600000000002 2.4036900000000001]  ProductsOfInertiaUnits=kg*mm^2  BasedOnType=Density  Density=1000  DensityUnits=kg/(m^3)  DoExposeReferenceFrame=on  SerializedFrames=<Frames/>  GraphicType=FromGeometry  MarkerShape=Sphere  MarkerSize=10  MarkerSizeUnits=m  GraphicVisPropType=SimpleVisualProperties  GraphicDiffuseColor=[0.898039 0.917647 0.929412]  GraphicSpecularColor=[0.5 0.5 0.5 1.0]  GraphicAmbientColor=[0.15 0.15 0.15 1.0]  GraphicEmissiveColor=[0.0 0.0 0.0 1.0]  GraphicShininess=75  GraphicOpacity=1
  F : PMIOPort  Side=Left
  connections:
  F/RConn1 -- ReferenceFrame/RConn1 -- Solid/RConn1

== system Table_airbus_v1/Modèle mécanique/Table/table_1_RIGID/x15060_M_01002_Ens_cadre_Default_1_RIGID/x15060_M_01005_Ens_barre_de_cadre_2_Default_2_RIGID/x15060_M_01042_Barre_transversale_AA_DEFAULT_1_RIGID ==
  ReferenceFrame : sm_lib/Frames and Transforms/Reference Frame
  Solid : sm_lib/Body Elements/File Solid  ExtGeomFileName=15060-M-01042-Barre transversale_AA - DEFAULT_Défaut_sldprt.STL  UnitType=Custom  ExtGeomFileUnits=mm  StepReaderType=HEX  ExportConvexHullGeometry=off  InertiaType=Custom  Mass=0.60250400000000004  MassUnits=kg  CenterOfMass=[0 0 -1.04198e-12]  CenterOfMassUnits=mm  MomentsOfInertia=[20808.599999999999 20753.200000000001 65.337600000000009]  MomentsOfInertiaUnits=kg*mm^2  ProductsOfInertia=[0 0 0]  ProductsOfInertiaUnits=kg*mm^2  BasedOnType=Density  Density=1000  DensityUnits=kg/(m^3)  DoExposeReferenceFrame=on  SerializedFrames=<Frames/>  GraphicType=FromGeometry  MarkerShape=Sphere  MarkerSize=10  MarkerSizeUnits=m  GraphicVisPropType=SimpleVisualProperties  GraphicDiffuseColor=[0.898039 0.917647 0.929412]  GraphicSpecularColor=[0.5 0.5 0.5 1.0]  GraphicAmbientColor=[0.15 0.15 0.15 1.0]  GraphicEmissiveColor=[0.0 0.0 0.0 1.0]  GraphicShininess=75  GraphicOpacity=1
  F : PMIOPort  Side=Left
  connections:
  F/RConn1 -- ReferenceFrame/RConn1 -- Solid/RConn1

== system Table_airbus_v1/Modèle mécanique/Table/table_1_RIGID/x15060_M_01002_Ens_cadre_Default_1_RIGID/x15060_M_01005_Ens_barre_de_cadre_2_Default_2_RIGID/x15060_M_01043_Bride_de_barre_AA_DEFAULT_1_RIGID ==
  ReferenceFrame : sm_lib/Frames and Transforms/Reference Frame
  Solid : sm_lib/Body Elements/File Solid  ExtGeomFileName=15060-M-01043-Bride de barre_AA - DEFAULT_Défaut_sldprt.STL  UnitType=Custom  ExtGeomFileUnits=mm  StepReaderType=HEX  ExportConvexHullGeometry=off  InertiaType=Custom  Mass=0.0646534  MassUnits=kg  CenterOfMass=[0 -0.40050599999999997 5.0587200000000001]  CenterOfMassUnits=mm  MomentsOfInertia=[5.7510300000000001 34.636699999999998 39.315600000000003]  MomentsOfInertiaUnits=kg*mm^2  ProductsOfInertia=[0.038467100000000004 0 0]  ProductsOfInertiaUnits=kg*mm^2  BasedOnType=Density  Density=1000  DensityUnits=kg/(m^3)  DoExposeReferenceFrame=on  SerializedFrames=<Frames/>  GraphicType=FromGeometry  MarkerShape=Sphere  MarkerSize=10  MarkerSizeUnits=m  GraphicVisPropType=SimpleVisualProperties  GraphicDiffuseColor=[0.898039 0.917647 0.929412]  GraphicSpecularColor=[0.5 0.5 0.5 1.0]  GraphicAmbientColor=[0.15 0.15 0.15 1.0]  GraphicEmissiveColor=[0.0 0.0 0.0 1.0]  GraphicShininess=75  GraphicOpacity=1
  F : PMIOPort  Side=Left
  connections:
  F/RConn1 -- ReferenceFrame/RConn1 -- Solid/RConn1

== system Table_airbus_v1/Modèle mécanique/Table/table_1_RIGID/x15060_M_01002_Ens_cadre_Default_1_RIGID/x15060_M_01005_Ens_barre_de_cadre_2_Default_2_RIGID/x15060_M_01043_Bride_de_barre_AA_DEFAULT_2_RIGID ==
  ReferenceFrame : sm_lib/Frames and Transforms/Reference Frame
  Solid : sm_lib/Body Elements/File Solid  ExtGeomFileName=15060-M-01043-Bride de barre_AA - DEFAULT_Défaut_sldprt.STL  UnitType=Custom  ExtGeomFileUnits=mm  StepReaderType=HEX  ExportConvexHullGeometry=off  InertiaType=Custom  Mass=0.0646534  MassUnits=kg  CenterOfMass=[0 -0.40050599999999997 5.0587200000000001]  CenterOfMassUnits=mm  MomentsOfInertia=[5.7510300000000001 34.636699999999998 39.315600000000003]  MomentsOfInertiaUnits=kg*mm^2  ProductsOfInertia=[0.038467100000000004 0 0]  ProductsOfInertiaUnits=kg*mm^2  BasedOnType=Density  Density=1000  DensityUnits=kg/(m^3)  DoExposeReferenceFrame=on  SerializedFrames=<Frames/>  GraphicType=FromGeometry  MarkerShape=Sphere  MarkerSize=10  MarkerSizeUnits=m  GraphicVisPropType=SimpleVisualProperties  GraphicDiffuseColor=[0.898039 0.917647 0.929412]  GraphicSpecularColor=[0.5 0.5 0.5 1.0]  GraphicAmbientColor=[0.15 0.15 0.15 1.0]  GraphicEmissiveColor=[0.0 0.0 0.0 1.0]  GraphicShininess=75  GraphicOpacity=1
  F : PMIOPort  Side=Left
  connections:
  F/RConn1 -- ReferenceFrame/RConn1 -- Solid/RConn1

== system Table_airbus_v1/Modèle mécanique/Table/table_1_RIGID/x15060_M_01002_Ens_cadre_Default_1_RIGID/x15060_M_01005_Ens_barre_de_cadre_2_Default_2_RIGID/x15060_M_01053_Plaquette_haute_sur_glissiere_SYM_AA_DEFAULT_1_R ==
  ReferenceFrame : sm_lib/Frames and Transforms/Reference Frame
  Solid : sm_lib/Body Elements/File Solid  ExtGeomFileName=15060-M-01053-Plaquette haute sur glissiere - SYM_AA - DEFAULT_Défaut_sldprt.STL  UnitType=Custom  ExtGeomFileUnits=mm  StepReaderType=HEX  ExportConvexHullGeometry=off  InertiaType=Custom  Mass=0.16431999999999999  MassUnits=kg  CenterOfMass=[-0.632606 23.438800000000001 -4.9895300000000002]  CenterOfMassUnits=mm  MomentsOfInertia=[87.900800000000004 87.570599999999999 172.749]  MomentsOfInertiaUnits=kg*mm^2  ProductsOfInertia=[-0.0346886 0.044093199999999999 2.4038600000000003]  ProductsOfInertiaUnits=kg*mm^2  BasedOnType=Density  Density=1000  DensityUnits=kg/(m^3)  DoExposeReferenceFrame=on  SerializedFrames=<Frames/>  GraphicType=FromGeometry  MarkerShape=Sphere  MarkerSize=10  MarkerSizeUnits=m  GraphicVisPropType=SimpleVisualProperties  GraphicDiffuseColor=[0.898039 0.917647 0.929412]  GraphicSpecularColor=[0.5 0.5 0.5 1.0]  GraphicAmbientColor=[0.15 0.15 0.15 1.0]  GraphicEmissiveColor=[0.0 0.0 0.0 1.0]  GraphicShininess=75  GraphicOpacity=1
  F : PMIOPort  Side=Left
  connections:
  F/RConn1 -- ReferenceFrame/RConn1 -- Solid/RConn1

== system Table_airbus_v1/Modèle mécanique/Table/table_1_RIGID/x15060_M_01002_Ens_cadre_Default_1_RIGID/x15060_M_01005_Ens_barre_de_cadre_2_Default_2_RIGID/x15060_NLM_Goupille_cyl_3_Lgr_16_03320_03x16_AA_DEFAULT_1_RIGID ==
  ReferenceFrame : sm_lib/Frames and Transforms/Reference Frame
  Solid : sm_lib/Body Elements/File Solid  ExtGeomFileName=15060-NLM-Goupille cyl I3 Lgr 16 - 03320-03x16_AA - DEFAULT_Défaut_sldprt.STL  UnitType=Custom  ExtGeomFileUnits=mm  StepReaderType=HEX  ExportConvexHullGeometry=off  InertiaType=Custom  Mass=0.000113097  MassUnits=kg  CenterOfMass=[8 0 0]  CenterOfMassUnits=mm  MomentsOfInertia=[0.00012723500000000001 0.0024763599999999999 0.0024763599999999999]  MomentsOfInertiaUnits=kg*mm^2  ProductsOfInertia=[0 0 0]  ProductsOfInertiaUnits=kg*mm^2  BasedOnType=Density  Density=1000  DensityUnits=kg/(m^3)  DoExposeReferenceFrame=on  SerializedFrames=<Frames/>  GraphicType=FromGeometry  MarkerShape=Sphere  MarkerSize=10  MarkerSizeUnits=m  GraphicVisPropType=SimpleVisualProperties  GraphicDiffuseColor=[0.792157 0.819608 0.933333]  GraphicSpecularColor=[0.5 0.5 0.5 1.0]  GraphicAmbientColor=[0.15 0.15 0.15 1.0]  GraphicEmissiveColor=[0.0 0.0 0.0 1.0]  GraphicShininess=75  GraphicOpacity=1
  F : PMIOPort  Side=Left
  connections:
  F/RConn1 -- Solid/RConn1 -- ReferenceFrame/RConn1

== system Table_airbus_v1/Modèle mécanique/Table/table_1_RIGID/x15060_M_01002_Ens_cadre_Default_1_RIGID/x15060_M_01005_Ens_barre_de_cadre_2_Default_2_RIGID/x15060_NLM_Goupille_cyl_3_Lgr_16_03320_03x16_AA_DEFAULT_2_RIGID ==
  ReferenceFrame : sm_lib/Frames and Transforms/Reference Frame
  Solid : sm_lib/Body Elements/File Solid  ExtGeomFileName=15060-NLM-Goupille cyl I3 Lgr 16 - 03320-03x16_AA - DEFAULT_Défaut_sldprt.STL  UnitType=Custom  ExtGeomFileUnits=mm  StepReaderType=HEX  ExportConvexHullGeometry=off  InertiaType=Custom  Mass=0.000113097  MassUnits=kg  CenterOfMass=[8 0 0]  CenterOfMassUnits=mm  MomentsOfInertia=[0.00012723500000000001 0.0024763599999999999 0.0024763599999999999]  MomentsOfInertiaUnits=kg*mm^2  ProductsOfInertia=[0 0 0]  ProductsOfInertiaUnits=kg*mm^2  BasedOnType=Density  Density=1000  DensityUnits=kg/(m^3)  DoExposeReferenceFrame=on  SerializedFrames=<Frames/>  GraphicType=FromGeometry  MarkerShape=Sphere  MarkerSize=10  MarkerSizeUnits=m  GraphicVisPropType=SimpleVisualProperties  GraphicDiffuseColor=[0.792157 0.819608 0.933333]  GraphicSpecularColor=[0.5 0.5 0.5 1.0]  GraphicAmbientColor=[0.15 0.15 0.15 1.0]  GraphicEmissiveColor=[0.0 0.0 0.0 1.0]  GraphicShininess=75  GraphicOpacity=1
  F : PMIOPort  Side=Left
  connections:
  F/RConn1 -- Solid/RConn1 -- ReferenceFrame/RConn1

== system Table_airbus_v1/Modèle mécanique/Table/table_1_RIGID/x15060_M_01002_Ens_cadre_Default_1_RIGID/x15060_M_01005_Ens_barre_de_cadre_2_Default_2_RIGID/x15060_NLM_Poign_e_Miniwing_M6_06652_006_X_15_1_RIGID ==
  ReferenceFrame : sm_lib/Frames and Transforms/Reference Frame
  Solid : sm_lib/Body Elements/File Solid  ExtGeomFileName=15060-NLM-Poignee Miniwing M6 - 06652-006 X 15_Défaut_sldprt.STL  UnitType=Custom  ExtGeomFileUnits=mm  StepReaderType=HEX  ExportConvexHullGeometry=off  InertiaType=Custom  Mass=0.0031415499999999999  MassUnits=kg  CenterOfMass=[0 5.4933500000000004 0]  CenterOfMassUnits=mm  MomentsOfInertia=[0.151592 0.116684 0.22078500000000001]  MomentsOfInertiaUnits=kg*mm^2  ProductsOfInertia=[0 0.0064548499999999998 0]  ProductsOfInertiaUnits=kg*mm^2  BasedOnType=Density  Density=1000  DensityUnits=kg/(m^3)  DoExposeReferenceFrame=on  SerializedFrames=<Frames/>  GraphicType=FromGeometry  MarkerShape=Sphere  MarkerSize=10  MarkerSizeUnits=m  GraphicVisPropType=SimpleVisualProperties  GraphicDiffuseColor=[0.792157 0.819608 0.933333]  GraphicSpecularColor=[0.5 0.5 0.5 1.0]  GraphicAmbientColor=[0.15 0.15 0.15 1.0]  GraphicEmissiveColor=[0.0 0.0 0.0 1.0]  GraphicShininess=75  GraphicOpacity=1
  F : PMIOPort  Side=Left
  connections:
  F/RConn1 -- Solid/RConn1 -- ReferenceFrame/RConn1

== system Table_airbus_v1/Modèle mécanique/Table/table_1_RIGID/x15060_M_01002_Ens_cadre_Default_1_RIGID/x15060_M_01005_Ens_barre_de_cadre_2_Default_2_RIGID/x15060_NLM_Poign_e_Miniwing_M6_06652_006_X_15_2_RIGID ==
  ReferenceFrame : sm_lib/Frames and Transforms/Reference Frame
  Solid : sm_lib/Body Elements/File Solid  ExtGeomFileName=15060-NLM-Poignee Miniwing M6 - 06652-006 X 15_Défaut_sldprt.STL  UnitType=Custom  ExtGeomFileUnits=mm  StepReaderType=HEX  ExportConvexHullGeometry=off  InertiaType=Custom  Mass=0.0031415499999999999  MassUnits=kg  CenterOfMass=[0 5.4933500000000004 0]  CenterOfMassUnits=mm  MomentsOfInertia=[0.151592 0.116684 0.22078500000000001]  MomentsOfInertiaUnits=kg*mm^2  ProductsOfInertia=[0 0.0064548499999999998 0]  ProductsOfInertiaUnits=kg*mm^2  BasedOnType=Density  Density=1000  DensityUnits=kg/(m^3)  DoExposeReferenceFrame=on  SerializedFrames=<Frames/>  GraphicType=FromGeometry  MarkerShape=Sphere  MarkerSize=10  MarkerSizeUnits=m  GraphicVisPropType=SimpleVisualProperties  GraphicDiffuseColor=[0.792157 0.819608 0.933333]  GraphicSpecularColor=[0.5 0.5 0.5 1.0]  GraphicAmbientColor=[0.15 0.15 0.15 1.0]  GraphicEmissiveColor=[0.0 0.0 0.0 1.0]  GraphicShininess=75  GraphicOpacity=1
  F : PMIOPort  Side=Left
  connections:
  F/RConn1 -- Solid/RConn1 -- ReferenceFrame/RConn1

== system Table_airbus_v1/Modèle mécanique/Table/table_1_RIGID/x15060_M_01002_Ens_cadre_Default_1_RIGID/x15060_M_01005_Ens_barre_de_cadre_2_Default_2_RIGID/x15060_Rondelle_Rondelle_Etroite_Z_4_1_RIGID ==
  ReferenceFrame : sm_lib/Frames and Transforms/Reference Frame
  Solid : sm_lib/Body Elements/File Solid  ExtGeomFileName=15060-Rondelle-_Rondelle Etroite Z 4_Défaut_sldprt.STL  UnitType=Custom  ExtGeomFileUnits=mm  StepReaderType=HEX  ExportConvexHullGeometry=off  InertiaType=Custom  Mass=3.9276200000000002e-05  MassUnits=kg  CenterOfMass=[0 0.40000000000000002 0]  CenterOfMassUnits=mm  MomentsOfInertia=[0.000246319 0.00048844899999999996 0.000246319]  MomentsOfInertiaUnits=kg*mm^2  ProductsOfInertia=[0 0 0]  ProductsOfInertiaUnits=kg*mm^2  BasedOnType=Density  Density=1000  DensityUnits=kg/(m^3)  DoExposeReferenceFrame=on  SerializedFrames=<Frames/>  GraphicType=FromGeometry  MarkerShape=Sphere  MarkerSize=10  MarkerSizeUnits=m  GraphicVisPropType=SimpleVisualProperties  GraphicDiffuseColor=[0.792157 0.819608 0.933333]  GraphicSpecularColor=[0.5 0.5 0.5 1.0]  GraphicAmbientColor=[0.15 0.15 0.15 1.0]  GraphicEmissiveColor=[0.0 0.0 0.0 1.0]  GraphicShininess=75  GraphicOpacity=1
  F : PMIOPort  Side=Left
  connections:
  F/RConn1 -- ReferenceFrame/RConn1 -- Solid/RConn1

== system Table_airbus_v1/Modèle mécanique/Table/table_1_RIGID/x15060_M_01002_Ens_cadre_Default_1_RIGID/x15060_M_01005_Ens_barre_de_cadre_2_Default_2_RIGID/x15060_Rondelle_Rondelle_Etroite_Z_4_2_RIGID ==
  ReferenceFrame : sm_lib/Frames and Transforms/Reference Frame
  Solid : sm_lib/Body Elements/File Solid  ExtGeomFileName=15060-Rondelle-_Rondelle Etroite Z 4_Défaut_sldprt.STL  UnitType=Custom  ExtGeomFileUnits=mm  StepReaderType=HEX  ExportConvexHullGeometry=off  InertiaType=Custom  Mass=3.9276200000000002e-05  MassUnits=kg  CenterOfMass=[0 0.40000000000000002 0]  CenterOfMassUnits=mm  MomentsOfInertia=[0.000246319 0.00048844899999999996 0.000246319]  MomentsOfInertiaUnits=kg*mm^2  ProductsOfInertia=[0 0 0]  ProductsOfInertiaUnits=kg*mm^2  BasedOnType=Density  Density=1000  DensityUnits=kg/(m^3)  DoExposeReferenceFrame=on  SerializedFrames=<Frames/>  GraphicType=FromGeometry  MarkerShape=Sphere  MarkerSize=10  MarkerSizeUnits=m  GraphicVisPropType=SimpleVisualProperties  GraphicDiffuseColor=[0.792157 0.819608 0.933333]  GraphicSpecularColor=[0.5 0.5 0.5 1.0]  GraphicAmbientColor=[0.15 0.15 0.15 1.0]  GraphicEmissiveColor=[0.0 0.0 0.0 1.0]  GraphicShininess=75  GraphicOpacity=1
  F : PMIOPort  Side=Left
  connections:
  F/RConn1 -- ReferenceFrame/RConn1 -- Solid/RConn1

== system Table_airbus_v1/Modèle mécanique/Table/table_1_RIGID/x15060_M_01002_Ens_cadre_Default_1_RIGID/x15060_M_01005_Ens_barre_de_cadre_2_Default_2_RIGID/x15060_Rondelle_Rondelle_Etroite_Z_4_3_RIGID ==
  ReferenceFrame : sm_lib/Frames and Transforms/Reference Frame
  Solid : sm_lib/Body Elements/File Solid  ExtGeomFileName=15060-Rondelle-_Rondelle Etroite Z 4_Défaut_sldprt.STL  UnitType=Custom  ExtGeomFileUnits=mm  StepReaderType=HEX  ExportConvexHullGeometry=off  InertiaType=Custom  Mass=3.9276200000000002e-05  MassUnits=kg  CenterOfMass=[0 0.40000000000000002 0]  CenterOfMassUnits=mm  MomentsOfInertia=[0.000246319 0.00048844899999999996 0.000246319]  MomentsOfInertiaUnits=kg*mm^2  ProductsOfInertia=[0 0 0]  ProductsOfInertiaUnits=kg*mm^2  BasedOnType=Density  Density=1000  DensityUnits=kg/(m^3)  DoExposeReferenceFrame=on  SerializedFrames=<Frames/>  GraphicType=FromGeometry  MarkerShape=Sphere  MarkerSize=10  MarkerSizeUnits=m  GraphicVisPropType=SimpleVisualProperties  GraphicDiffuseColor=[0.792157 0.819608 0.933333]  GraphicSpecularColor=[0.5 0.5 0.5 1.0]  GraphicAmbientColor=[0.15 0.15 0.15 1.0]  GraphicEmissiveColor=[0.0 0.0 0.0 1.0]  GraphicShininess=75  GraphicOpacity=1
  F : PMIOPort  Side=Left
  connections:
  F/RConn1 -- ReferenceFrame/RConn1 -- Solid/RConn1
